simulink model "CSK_Std_PulseTrain_SM2015b_Attempt3"  (R2015b)
settings: Solver=ode23s  StartTime=0.0  StopTime=800  RelTol=1e-12
values from neighbouring files (symbols this model uses):
  beta = 25.6    [RUN_021317.m]    (also in RUN_021417.m; RUN_022117.m)
  delay = 0    [RUN_022117.m]
  freq = message baud rate    [ErrChk.m]    (also in LoadText.m = Message Frequency; ProcessSync.m = expected bit frequency; ProcessSyncPeak.m = expected bit frequency; ProcessSyncPeak2.m = expected bit frequency)
  rho = 2    [RUN_021317.m]    (also in RUN_021417.m; RUN_022117.m)
  sig = 10    [RUN_021317.m]    (also in RUN_021417.m; RUN_022117.m)
  x0 = [.1,.2,.3]    [RUN_021317.m]    (also in RUN_021417.m; RUN_022117.m)
  z0 = x0    [RUN_021317.m]    (also in RUN_021417.m; RUN_022117.m)
settings Model: Creator=Dan  LastModifiedBy=dbrown63
settings DataIOCC: SaveFormat=Array
settings DebuggingCC: SolverPrmCheckMsg=warning  AllowSymbolicDim=on
settings HardwareCC: ProdBitPerPointer=32  ProdLargestAtomicFloat=None  ProdIntDivRoundTo=Undefined  ProdEndianess=Unspecified  ProdWordSize=32  ProdHWDeviceType=32-bit Generic
settings GRTTargetCC: GeneratePreprocessorConditionals=Disable all
settings ConfigComp: CovModelRefEnable=Off  CovSFcnEnable=off

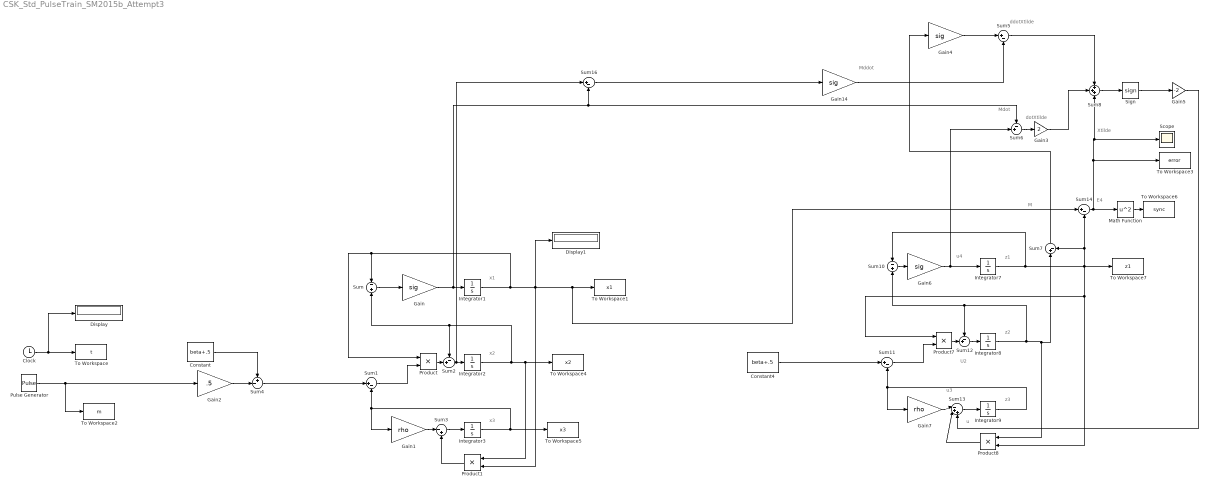
== system CSK_Std_PulseTrain_SM2015b_Attempt3 ==
  note: ddotXtilde
  note: Mddot
  note: Xtilde
  note: dotXtilde
  note: Mdot
  note: u
  note: M
  note: E4
  note: u3
  note: U2
  note: u4
  note: x1
  note: x2
  note: x3
  note: z1
  note: z2
  note: z3
  Clock : Clock
  Constant : Constant  Value=beta+.5
  Constant4 : Constant  Value=beta+.5
  Display : Display
      settings: Decimation=5
  Display1 : Display
      settings: Decimation=5
  Gain{,4,6,14} (4 alike) : Gain  Gain=sig
  Gain1 : Gain  Gain=rho
  Gain2 : Gain  Gain=.5
  Gain3 : Gain  Gain=2
  Gain5 : Gain  Gain=-2
  Gain7 : Gain  Gain=rho
  Integrator1 : Integrator  InitialCondition=x0(1)
  Integrator2 : Integrator  InitialCondition=x0(2)
  Integrator3 : Integrator  InitialCondition=x0(3)
  Integrator7 : Integrator  InitialCondition=z0(1)
  Integrator8 : Integrator  InitialCondition=z0(2)
  Integrator9 : Integrator  InitialCondition=z0(3)
  Math Function : Math  Operator=square  SaturateOnIntegerOverflow=on
  Product{,1,7..8} (4 alike) : Product
  Pulse Generator : DiscretePulseGenerator  PulseType=Time based  Period=2/freq  PulseWidth=50  PhaseDelay=delay
  Scope : Scope
  Sign : Signum  ZeroCross=off
  Sum : Sum  Inputs=-|+
  Sum{1,5,7,11,14,16} (6 alike) : Sum  Inputs=|+-
  Sum10 : Sum  Inputs=-|+
  Sum12 : Sum  Inputs=-+|
  Sum13 : Sum  Inputs=|-++
  Sum2 : Sum  Inputs=-+|
  Sum3 : Sum  Inputs=|-+
  Sum4 : Sum  Inputs=+-|
  Sum6 : Sum  Inputs=-+|
  Sum8 : Sum  Inputs=+++
  To Workspace : ToWorkspace  VariableName=t  SampleTime=-1
  To Workspace1 : ToWorkspace  VariableName=x1  SampleTime=-1
  To Workspace2 : ToWorkspace  VariableName=m  SampleTime=-1
  To Workspace3 : ToWorkspace  VariableName=error  SampleTime=-1
  To Workspace4 : ToWorkspace  VariableName=x2  SampleTime=-1
  To Workspace5 : ToWorkspace  VariableName=x3  SampleTime=-1
  To Workspace6 : ToWorkspace  VariableName=sync  SampleTime=-1
  To Workspace7 : ToWorkspace  VariableName=z1  SampleTime=-1
  wires:
  Sum/1 -> Gain/1
  Sum1/1 -> Product/2
  Integrator3/1 -> To Workspace5/1, Gain1/1, Sum1/2
  Sum3/1 -> Integrator3/1
  Product1/1 -> Sum3/2
  Integrator2/1 -> To Workspace4/1, Product1/1, Sum2/1, Sum/2
  Gain1/1 -> Sum3/1
  Gain2/1 -> Sum4/2
  Constant/1 -> Sum4/1
  Sum4/1 -> Sum1/1
  Clock/1 -> Display/1, To Workspace/1
  Product/1 -> Sum2/2
  Sum2/1 -> Sum16/1, Integrator2/1
  Pulse Generator/1 -> To Workspace2/1, Gain2/1
  Sum10/1 -> Gain6/1
  Sum11/1 -> Product7/2
  Sum13/1 -> Integrator9/1
  Product7/1 -> Sum12/2
  Sum12/1 -> Integrator8/1
  Sum14/1 -> Scope/1, Sum8/3, To Workspace3/1, Math Function/1
  Integrator1/1 -> Sum/1, Product/1, Product1/2, Display1/1, Sum14/1, To Workspace1/1
  Math Function/1 -> To Workspace6/1
  Gain6/1 -> Sum6/2, Integrator7/1
  Integrator8/1 -> Sum7/1, Product8/1, Sum12/1, Sum10/2
  Gain7/1 -> Sum13/1
  Product8/1 -> Sum13/2
  Integrator9/1 -> Gain7/1, Sum11/2
  Gain/1 -> Sum6/1, Sum16/2, Integrator1/1
  Constant4/1 -> Sum11/1
  Integrator7/1 -> Product7/1, Product8/2, To Workspace7/1, Sum7/2, Sum14/2, Sum10/1
  Sum16/1 -> Gain14/1
  Sum6/1 -> Gain3/1
  Gain14/1 -> Sum5/2
  Gain4/1 -> Sum5/1
  Sum7/1 -> Gain4/1
  Gain3/1 -> Sum8/2
  Sum5/1 -> Sum8/1
  Sum8/1 -> Sign/1
  Sign/1 -> Gain5/1
  Gain5/1 -> Sum13/3
